simulink model "LRN"  (R2024b)
settings: Solver=FixedStepDiscrete  StartTime=0.0  StopTime=1  RelTol=1e-3
settings Model: DataTypeOverride=Off  Creator=valen  LastModifiedBy=valen
settings SolverCC: AlgebraicLoopSolver=TrustRegion
settings DataIOCC: LimitDataPoints=on  SaveOutput=off  SaveTime=off
settings OptimizationCC: BlockReduction=off  ConditionallyExecuteInputs=off  DefaultParameterBehavior=Inlined  LifeSpan=inf
settings DebuggingCC: AlgebraicLoopMsg=error  SingleTaskRateTransMsg=error  UnconnectedInputMsg=warning  UnconnectedOutputMsg=warning  UnconnectedLineMsg=warning  AllowSymbolicDim=off  StrictBusMsg=ErrorOnBusTreatedAsVector  SFUnexpectedBacktrackingDiag=warning  SFNoUnconditionalDefaultTransitionDiag=warning  SFExecutionAtInitializationDiag=none  ArithmeticOperatorsInVariantConditions=warning
settings HardwareCC: ProdBitPerPointer=32  ProdBitPerSizeT=32  ProdBitPerPtrDiffT=32  ProdLargestAtomicFloat=None  ProdIntDivRoundTo=Undefined  ProdEndianess=Unspecified  ProdWordSize=32  ProdHWDeviceType=ASIC/FPGA->ASIC/FPGA  ProdEqTarget=off
settings ModelReferenceCC: EnableRefExpFcnMdlSchedulingChecks=on
settings SFSimCC: SimUseLocalCustomCode=off  CustomCodeUndefinedFunction=UseInterfaceOnly
settings RTWCC: RTWUseLocalCustomCode=off  GPUComputeCapability=3.5
settings CodeAppCC: StateflowObjectComments=on
settings GRTTargetCC: TargetLangStandard=C89/C90 (ANSI)
settings ConfigComp: CovScope=ReferencedModels  CovMetricSettings=dw  CovSaveCumulativeToWorkspaceVar=on  CovSaveSingleToWorkspaceVar=on  CovExternalEMLEnable=off  CovSFcnEnable=off

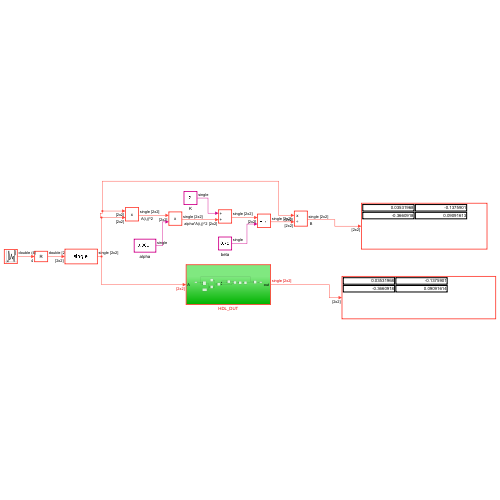
[thumbnail: Simulink's stored preview of the top-level diagram]
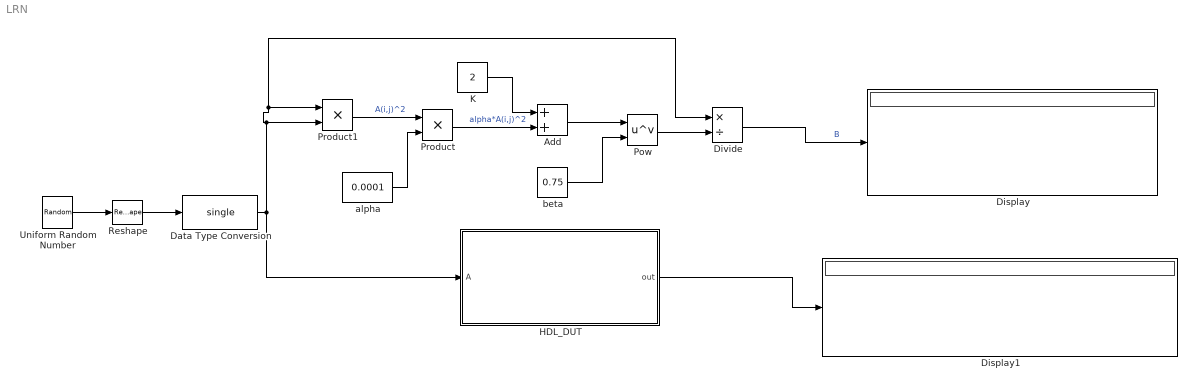
== system LRN ==
  Add : Sum
  Data Type Conversion : DataTypeConversion  OutDataTypeStr=single  SaturateOnIntegerOverflow=off  RndMeth=Floor
  Display : Display
  Display1 : Display
  Divide : Product  Inputs=*/  RndMeth=Zero  SaturateOnIntegerOverflow=on
  HDL_DUT : Subsystem
  K : Constant  Value=2  OutDataTypeStr=single
  Pow : Math  Operator=pow  SignedPower=on  RndMeth=Zero
  Product : Product  OutDataTypeStr=single
  Product1 : Product
  Reshape : Reshape  OutputDimensionality=Customize  OutputDimensions=[2,2]
  Uniform Random Number : UniformRandomNumber  Seed=[0;1;2;3]  SampleTime=0.1
  alpha : Constant  Value=0.0001  OutDataTypeStr=single
  beta : Constant  Value=0.75  OutDataTypeStr=single
  wires:
  Uniform Random Number/1 -> Reshape/1
  Reshape/1 -> Data Type Conversion/1
  Pow/1 -> Divide/2
  Product/1 -> Add/2  "alpha*A(i,j)^2"
  alpha/1 -> Product/2
  Product1/1 -> Product/1  "A(i,j)^2"
  beta/1 -> Pow/2
  Add/1 -> Pow/1
  K/1 -> Add/1
  Divide/1 -> Display/1  "B"
  HDL_DUT/1(out) -> Display1/1
  Data Type Conversion/1 -> HDL_DUT/1(A), Product1/2, Divide/1, Product1/1

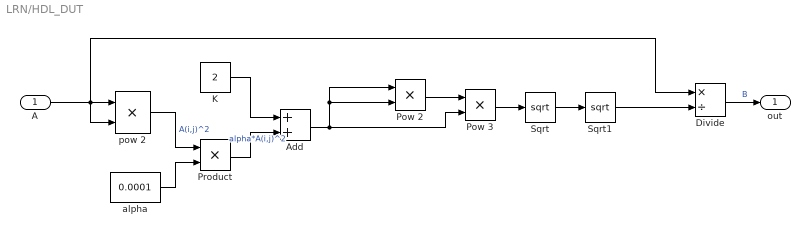
== system LRN/HDL_DUT ==
  A : Inport
  Add : Sum
  Divide : Product  Inputs=*/  RndMeth=Zero  SaturateOnIntegerOverflow=on
  K : Constant  Value=2  OutDataTypeStr=single
  Pow 2 : Product
  Pow 3 : Product
  Product : Product
  Sqrt : Sqrt
  Sqrt1 : Sqrt  OutDataTypeStr=Inherit: Inherit via internal rule
  alpha : Constant  Value=0.0001  OutDataTypeStr=single
  pow 2 : Product  InputSameDT=on
  out : Outport  VectorParamsAs1DForOutWhenUnconnected=off
  wires:
  pow 2/1 -> Product/1  "A(i,j)^2"
  alpha/1 -> Product/2
  Product/1 -> Add/2  "alpha*A(i,j)^2"
  K/1 -> Add/1
  Add/1 -> Pow 3/2, Pow 2/2, Pow 2/1
  Divide/1 -> out/1  "B"
  Pow 2/1 -> Pow 3/1
  Pow 3/1 -> Sqrt/1
  Sqrt/1 -> Sqrt1/1
  A/1 -> pow 2/2, Divide/1, pow 2/1
  Sqrt1/1 -> Divide/2
